simulink model "ex00_model"  (R2023a)
settings: Solver=FixedStepDiscrete  StartTime=0.0  StopTime=1  RelTol=1e-3
values from neighbouring files (symbols this model uses):
  E0 = E(1,:)    [ex00_config.m]
  E1 = E(2,:)    [ex00_config.m]
  E2 = E(3,:)    [ex00_config.m]
  E3 = E(4,:)    [ex00_config.m]
  Fc = 125e3    (= 125000)    [ex00_config.m]
  fir_num = fir1(fir_ord, Wn, hann(fir_ord+1))    [ex00_config.m]
  L = 4    [ex00_config.m]
  Ts = 1/Fs    (= 1e-06)    [ex00_config.m]
libraries: dspsigops x5, dspsrcs4 x2
settings Model: Creator=daniele  LastModifiedBy=daniele

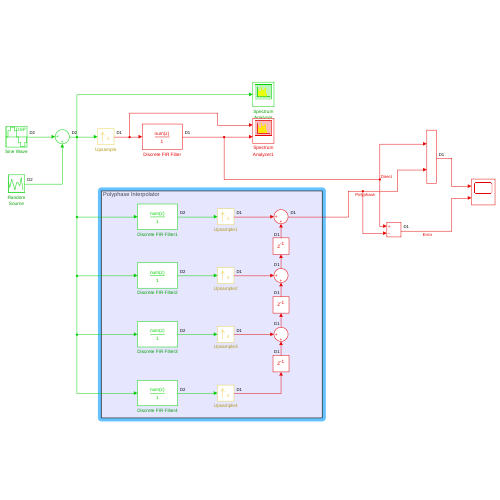
[thumbnail: Simulink's stored preview of the top-level diagram]
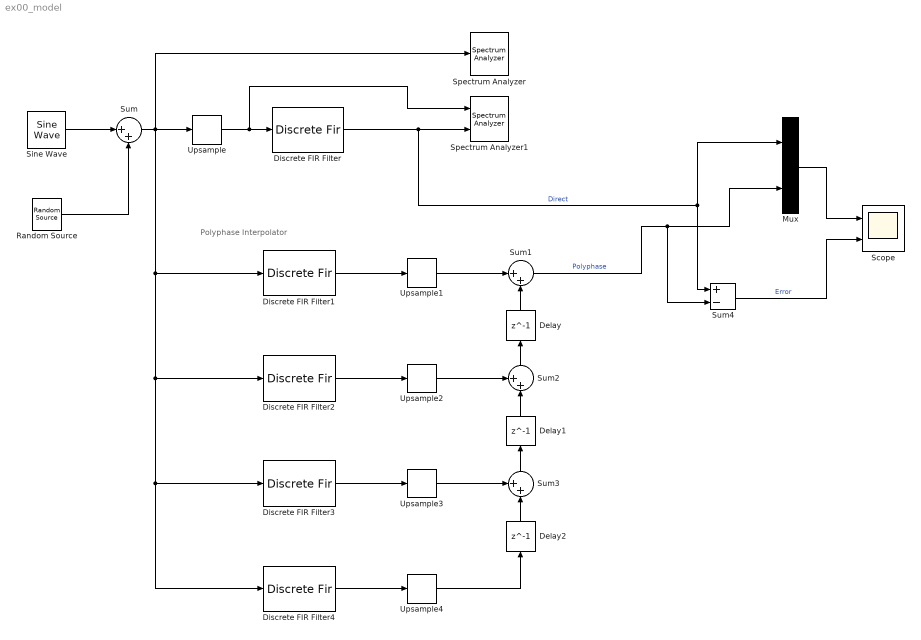
== system ex00_model ==
  note: Polyphase Interpolator
  Delay : Delay  DelayLength=1
  Delay1 : Delay  DelayLength=1
  Delay2 : Delay  DelayLength=1
  Discrete FIR Filter : DiscreteFir  Coefficients=fir_num
  Discrete FIR Filter1 : DiscreteFir  Coefficients=E0
  Discrete FIR Filter2 : DiscreteFir  Coefficients=E1
  Discrete FIR Filter3 : DiscreteFir  Coefficients=E2
  Discrete FIR Filter4 : DiscreteFir  Coefficients=E3
  Mux : Mux  Inputs=2
  Random Source : dspsrcs4/Random Source  SrcType=Gaussian  NormMethod=Ziggurat  CltLength=12  MinVal=0  MaxVal=1  MeanVal=0  VarVal=0.1  RepMode=Not repeatable  rawSeed=1  IsInherit=off  SampMode=Discrete  SampTime=Ts  SampFrame=1  DataType=Double  OutComplex=Real  OutputFrames=off
  Scope : Scope  NumInputPorts=2
  Sine Wave : dspsrcs4/Sine Wave  Amplitude=1  Frequency=Fc  Phase=pi/2  SampleMode=Discrete  OutComplex=Real  CompMethod=Trigonometric fcn  TableSize=Speed  SampleTime=Ts  SamplesPerFrame=1  ResetState=Restart at time zero  OutputFrames=off  dataType=double  wordLen=16  udDataType=sfix(16)  fracBitsMode=Best precision  numFracBits=15  OutDataTypeStr=double  LastOutDataTypeStr=double
  Spectrum Analyzer : SpectrumAnalyzer  WindowPosition=[99.000000,52.000000,800.000000,500.000000,]  Visible=on  ScopeFrameLocation=window  Span=1000000  StartFrequency=-500000  StopFrequency=500000  YLimits=[-21.41957255,27.72158598]  ColorLimits=[-20 80]  DefaultConfigurationName=spbscopes.SpectrumAnalyzerBlockCfg  IsFrequencyInputMode=0  FrequencyVectorPort=0  FrequencyVectorFromPort=0  FrequencyInputRBWPort=0  FrequencyInputRBWFromPort=0
  Spectrum Analyzer1 : SpectrumAnalyzer  NumInputPorts=2  WindowPosition=[225.000000,52.000000,800.000000,500.000000,]  Visible=on  ScopeFrameLocation=window  Span=4000000  StartFrequency=-2000000  StopFrequency=2000000  YLimits=[-167.85898637,31.8541331]  ColorLimits=[-20 80]  ShowLegend=on  DefaultConfigurationName=spbscopes.SpectrumAnalyzerBlockCfg  IsFrequencyInputMode=0  FrequencyVectorPort=0  FrequencyVectorFromPort=0  FrequencyInputRBWPort=0  FrequencyInputRBWFromPort=0
  Sum : Sum  Inputs=|++
  Sum1 : Sum  Inputs=|++
  Sum2 : Sum  Inputs=++|
  Sum3 : Sum  Inputs=++|
  Sum4 : Sum  Inputs=+-
  Upsample{,1..4} (5 alike) : dspsigops/Upsample  FactorSource=Dialog parameter  N=L  Nmax=16  phase=0  RateOptions=Allow multirate processing  ic=0  mode=Unused parameter value
      settings: LibrarySourceBlock=dsphdlsupportsigops/Upsample
  wires:
  Sine Wave/1 -> Sum/1
  Random Source/1 -> Sum/2
  Sum/1 -> Discrete FIR Filter4/1, Discrete FIR Filter3/1, Discrete FIR Filter2/1, Discrete FIR Filter1/1, Spectrum Analyzer/1, Upsample/1
  Upsample/1 -> Spectrum Analyzer1/1, Discrete FIR Filter/1
  Discrete FIR Filter/1 -> Mux/1, Sum4/1, Spectrum Analyzer1/2  "Direct"
  Discrete FIR Filter1/1 -> Upsample1/1
  Discrete FIR Filter2/1 -> Upsample2/1
  Discrete FIR Filter3/1 -> Upsample3/1
  Discrete FIR Filter4/1 -> Upsample4/1
  Upsample4/1 -> Delay2/1
  Delay2/1 -> Sum3/2
  Upsample3/1 -> Sum3/1
  Sum3/1 -> Delay1/1
  Delay1/1 -> Sum2/2
  Upsample2/1 -> Sum2/1
  Sum2/1 -> Delay/1
  Delay/1 -> Sum1/2
  Upsample1/1 -> Sum1/1
  Sum1/1 -> Mux/2, Sum4/2  "Polyphase"
  Sum4/1 -> Scope/2  "Error"
  Mux/1 -> Scope/1
